simulink model "microgrid_lcl"  (R2024b)
settings: Solver=ode4  StartTime=0.0  StopTime=0.1  FixedStep=5e-7  RelTol=1e-3
libraries: simulink x1
settings Model: Creator=muham  LastModifiedBy=muham
settings DataIOCC: SaveOutput=off

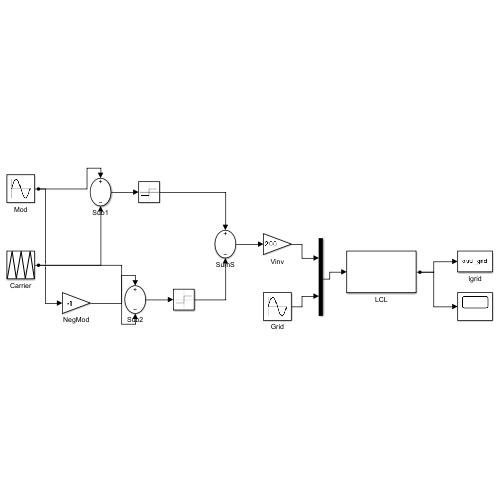
[thumbnail: Simulink's stored preview of the top-level diagram]
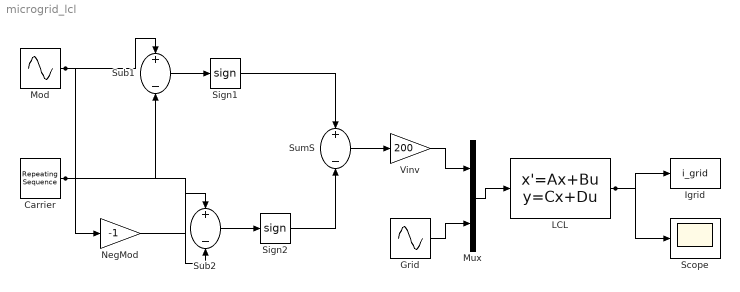
== system microgrid_lcl ==
  Carrier : simulink/Sources/Repeating Sequence  rep_seq_t=[0 5e-05 0.0001]  rep_seq_y=[0 1 0]
  Grid : Sin  Amplitude=325.2691  Frequency=376.9911  SampleTime=0
  Igrid : ToWorkspace  VariableName=i_grid  SaveFormat=Timeseries  SampleTime=-1
  LCL : StateSpace  A=[-1643.67816091954 1643.67816091954 -1149.42528735632;3108.69565217391 -3108.69565217391 2173.91304347826;63816.2093171666 -63816.2093171666 0]  B=[1149.42528735632 0;0 -2173.91304347826;0 0]  C=[0 1 0]  D=[0 0]  InitialCondition=[0;0;0]
  Mod : Sin  Amplitude=0.8146  Frequency=376.9911  Phase=0.05917  SampleTime=0
  Mux : Mux  Inputs=2
  NegMod : Gain  Gain=-1
  Scope : Scope
  Sign1 : Signum
  Sign2 : Signum
  Sub1 : Sum  Inputs=+-
  Sub2 : Sum  Inputs=+-
  SumS : Sum  Inputs=+-
  Vinv : Gain  Gain=200
  wires:
  Mod/1 -> Sub1/1, NegMod/1
  Carrier/1 -> Sub1/2, Sub2/2
  NegMod/1 -> Sub2/1
  Sub1/1 -> Sign1/1
  Sub2/1 -> Sign2/1
  Sign1/1 -> SumS/1
  Sign2/1 -> SumS/2
  SumS/1 -> Vinv/1
  Vinv/1 -> Mux/1
  Grid/1 -> Mux/2
  Mux/1 -> LCL/1
  LCL/1 -> Igrid/1, Scope/1
